simulink library "SignalConditioning_lib"  (Simulink 7.2)
settings: Solver=ode45  SolverMode=SingleTasking  StartTime=0.0  StopTime=10.0  RelTol=1e-3
undefined symbols (not defined in the file or in its folder): ADC, MAG3TempComp, XACCEL, XGYRO, XMAG, YACCEL, YGYRO, YMAG, ZACCEL, ZGYRO, ZMAG
libraries: First_Order_Filter_lib x4, SignalConditioning_lib x3, simulink_extras x2, simulink x1
settings Model: Creator=amurch  LastModifiedBy=lgarbs

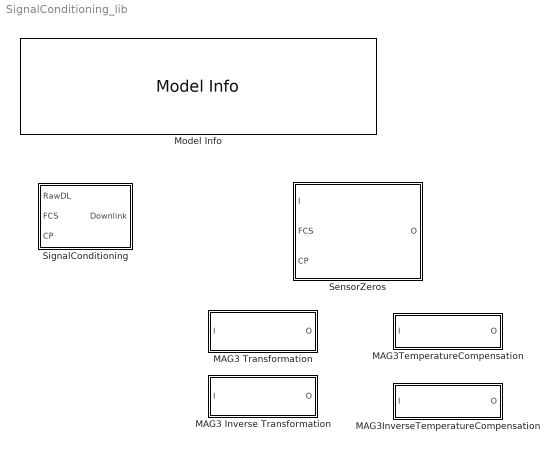
== system SignalConditioning_lib ==
  MAG3 Inverse Transformation : Subsystem
  MAG3 Transformation : Subsystem
  MAG3InverseTemperatureCompensation : Subsystem
  MAG3TemperatureCompensation : Subsystem
  Model Info : simulink/Model-Wide Utilities/Model Info  SystemSampleTime=-1  InitialBlockCM=None  BlockCM=None  Frame=on  DisplayStringWithTags=|  HorizontalTextAlignment=Center  LeftAlignmentValue=0.5  SourceBlockDiagram=SignalConditioning_lib  TagMaxNumber=20
      | Developed using Matlab Release 2007a
      | 
      | SVN:%<ModelVersion>
      | Last modifed by %<LastModifiedBy> on %<LastModificationDate>
  SensorZeros : Subsystem
  SignalConditioning : Subsystem

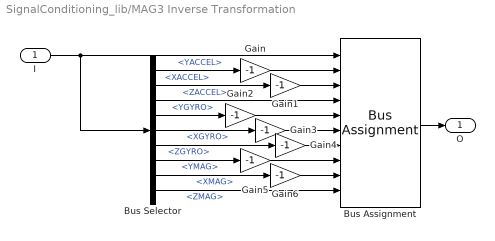
== system SignalConditioning_lib/MAG3 Inverse Transformation ==
  I : Inport  OutDataType=sfix(16)  OutScaling=2^0
  Bus Assignment : BusAssignment  AssignedSignals=XACCEL,YACCEL,ZACCEL,XGYRO,YGYRO,ZGYRO,XMAG,YMAG,ZMAG
  Bus Selector : BusSelector  OutputSignals=YACCEL,XACCEL,ZACCEL,YGYRO,XGYRO,ZGYRO,YMAG,XMAG,ZMAG
  Gain{,1..6} (7 alike) : Gain  Gain=-1  ParameterDataType=sfix(16)  ParameterScaling=2^0  OutDataType=sfix(16)  OutScaling=2^0
  O : Outport  OutDataType=sfix(16)  OutScaling=2^0
  wires:
  Bus Assignment/1 -> O/1
  I/1 -> Bus Assignment/1, Bus Selector/1
  Bus Selector/1 -> Gain/1  "<YACCEL>"
  Gain/1 -> Bus Assignment/2
  Bus Selector/2 -> Gain1/1  "<XACCEL>"
  Bus Selector/3 -> Bus Assignment/4  "<ZACCEL>"
  Gain2/1 -> Bus Assignment/5
  Gain3/1 -> Bus Assignment/6
  Bus Selector/4 -> Gain2/1  "<YGYRO>"
  Bus Selector/5 -> Gain3/1  "<XGYRO>"
  Bus Selector/6 -> Gain4/1  "<ZGYRO>"
  Gain5/1 -> Bus Assignment/8
  Bus Selector/7 -> Gain5/1  "<YMAG>"
  Bus Selector/8 -> Gain6/1  "<XMAG>"
  Bus Selector/9 -> Bus Assignment/10  "<ZMAG>"
  Gain1/1 -> Bus Assignment/3
  Gain4/1 -> Bus Assignment/7
  Gain6/1 -> Bus Assignment/9

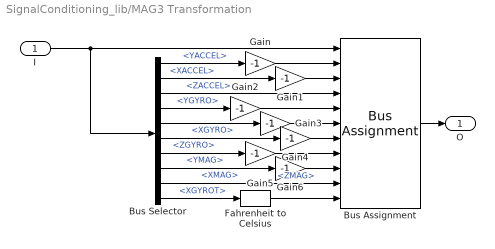
== system SignalConditioning_lib/MAG3 Transformation ==
  I : Inport  OutDataType=sfix(16)  OutScaling=2^0
  Bus Assignment : BusAssignment  AssignedSignals=ADC.XACCEL,ADC.YACCEL,ADC.ZACCEL,ADC.XGYRO,ADC.YGYRO,ADC.ZGYRO,ADC.XMAG,ADC.YMAG,ADC.ZMAG,ADC.XGYROT
  Bus Selector : BusSelector  OutputSignals=ADC.YACCEL,ADC.XACCEL,ADC.ZACCEL,ADC.YGYRO,ADC.XGYRO,ADC.ZGYRO,ADC.YMAG,ADC.XMAG,ADC.ZMAG,ADC.XGYROT
  Fahrenheit to Celsius : simulink_extras/Transformations/Fahrenheit to Celsius  SystemSampleTime=-1
  Gain{,1..6} (7 alike) : Gain  Gain=-1  ParameterDataType=sfix(16)  ParameterScaling=2^0  OutDataType=sfix(16)  OutScaling=2^0
  O : Outport  OutDataType=sfix(16)  OutScaling=2^0
  wires:
  Fahrenheit to Celsius/1 -> Bus Assignment/11
  Bus Selector/10 -> Fahrenheit to Celsius/1  "<XGYROT>"
  I/1 -> Bus Assignment/1, Bus Selector/1
  Bus Assignment/1 -> O/1
  Bus Selector/1 -> Gain/1  "<YACCEL>"
  Gain/1 -> Bus Assignment/2
  Bus Selector/2 -> Gain1/1  "<XACCEL>"
  Gain1/1 -> Bus Assignment/3
  Bus Selector/3 -> Bus Assignment/4  "<ZACCEL>"
  Gain2/1 -> Bus Assignment/5
  Gain3/1 -> Bus Assignment/6
  Bus Selector/4 -> Gain2/1  "<YGYRO>"
  Bus Selector/5 -> Gain3/1  "<XGYRO>"
  Gain4/1 -> Bus Assignment/7
  Bus Selector/6 -> Gain4/1  "<ZGYRO>"
  Gain5/1 -> Bus Assignment/8
  Gain6/1 -> Bus Assignment/9
  Bus Selector/7 -> Gain5/1  "<YMAG>"
  Bus Selector/8 -> Gain6/1  "<XMAG>"
  Bus Selector/9 -> Bus Assignment/10  "<ZMAG>"

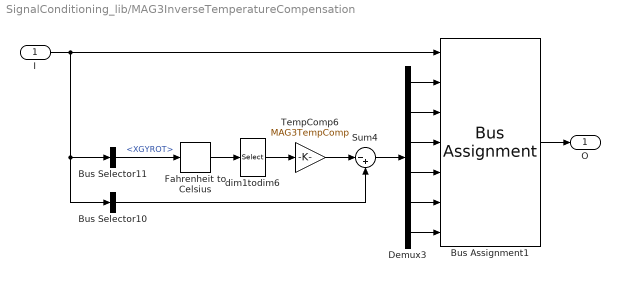
== system SignalConditioning_lib/MAG3InverseTemperatureCompensation ==
  I : Inport  OutDataType=sfix(16)  OutScaling=2^0
  Bus Assignment1 : BusAssignment  AssignedSignals=XGYRO,YGYRO,ZGYRO,XACCEL,YACCEL,ZACCEL
  Bus Selector10 : BusSelector  OutputSignals=XGYRO,YGYRO,ZGYRO,XACCEL,YACCEL,ZACCEL  OutputAsBus=on
  Bus Selector11 : BusSelector  OutputSignals=XGYROT
  Demux3 : Demux  Outputs=6
  Fahrenheit to Celsius : simulink_extras/Transformations/Fahrenheit to Celsius  SystemSampleTime=-1
  Sum4 : Sum  Inputs=|-+  OutDataType=sfix(16)  OutScaling=2^0
  TempComp6 : Gain  Gain=MAG3TempComp  ParameterDataType=sfix(16)  ParameterScaling=2^0  OutDataType=sfix(16)  OutScaling=2^0
  dim1todim6 : Selector  InputPortWidth=1  IndexOptions=Index vector (dialog)  Indices=[1 1 1 1 1 1]  OutputSizes=1
  O : Outport  OutDataType=sfix(16)  OutScaling=2^0
  wires:
  Bus Assignment1/1 -> O/1
  dim1todim6/1 -> TempComp6/1
  Sum4/1 -> Demux3/1
  Demux3/6 -> Bus Assignment1/7
  Demux3/5 -> Bus Assignment1/6
  Demux3/4 -> Bus Assignment1/5
  Demux3/3 -> Bus Assignment1/4
  Demux3/2 -> Bus Assignment1/3
  Demux3/1 -> Bus Assignment1/2
  Bus Selector10/1 -> Sum4/2
  TempComp6/1 -> Sum4/1
  Fahrenheit to Celsius/1 -> dim1todim6/1
  Bus Selector11/1 -> Fahrenheit to Celsius/1  "<XGYROT>"
  I/1 -> Bus Assignment1/1, Bus Selector11/1, Bus Selector10/1

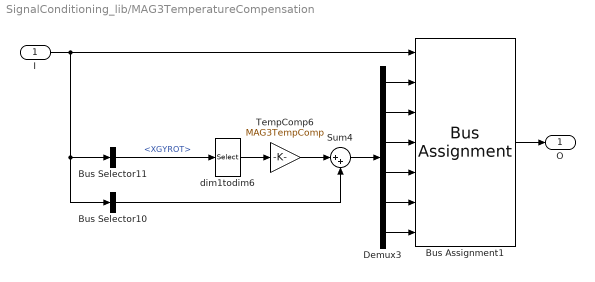
== system SignalConditioning_lib/MAG3TemperatureCompensation ==
  I : Inport  OutDataType=sfix(16)  OutScaling=2^0
  Bus Assignment1 : BusAssignment  AssignedSignals=ADC.XGYRO,ADC.YGYRO,ADC.ZGYRO,ADC.XACCEL,ADC.YACCEL,ADC.ZACCEL
  Bus Selector10 : BusSelector  OutputSignals=ADC.XGYRO,ADC.YGYRO,ADC.ZGYRO,ADC.XACCEL,ADC.YACCEL,ADC.ZACCEL  OutputAsBus=on
  Bus Selector11 : BusSelector  OutputSignals=ADC.XGYROT
  Demux3 : Demux  Outputs=6
  Sum4 : Sum  Inputs=|++  OutDataType=sfix(16)  OutScaling=2^0
  TempComp6 : Gain  Gain=MAG3TempComp  ParameterDataType=sfix(16)  ParameterScaling=2^0  OutDataType=sfix(16)  OutScaling=2^0
  dim1todim6 : Selector  InputPortWidth=1  IndexOptions=Index vector (dialog)  Indices=[1 1 1 1 1 1]  OutputSizes=1
  O : Outport  OutDataType=sfix(16)  OutScaling=2^0
  wires:
  I/1 -> Bus Selector10/1, Bus Selector11/1, Bus Assignment1/1
  Bus Selector11/1 -> dim1todim6/1  "<XGYROT>"
  TempComp6/1 -> Sum4/1
  Bus Selector10/1 -> Sum4/2
  Demux3/1 -> Bus Assignment1/2
  Demux3/2 -> Bus Assignment1/3
  Demux3/3 -> Bus Assignment1/4
  Demux3/4 -> Bus Assignment1/5
  Demux3/5 -> Bus Assignment1/6
  Demux3/6 -> Bus Assignment1/7
  Sum4/1 -> Demux3/1
  dim1todim6/1 -> TempComp6/1
  Bus Assignment1/1 -> O/1

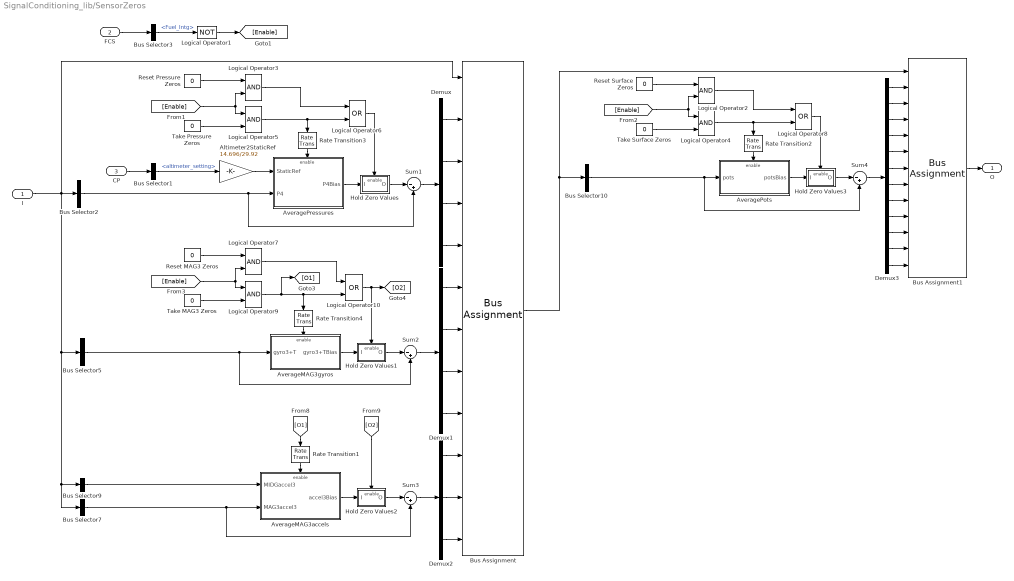
== system SignalConditioning_lib/SensorZeros ==
  I : Inport  OutDataType=sfix(16)  OutScaling=2^0
  FCS : Inport  Port=2  OutDataType=sfix(16)  OutScaling=2^0
  CP : Inport  Port=3  OutDataType=sfix(16)  OutScaling=2^0
  Altimeter2StaticRef : Gain  Gain=14.696/29.92  ParameterDataType=sfix(16)  ParameterScaling=2^0  OutDataType=sfix(16)  OutScaling=2^0
  AverageMAG3accels : Subsystem
  AverageMAG3gyros : Subsystem
  AveragePots : Subsystem
  AveragePressures : Subsystem
  Bus Assignment : BusAssignment  AssignedSignals=ADC.PSL,ADC.PDL,ADC.PSR,ADC.PDR,ADC.XGYRO,ADC.YGYRO,ADC.ZGYRO,ADC.XGYROT,ADC.XACCEL,ADC.YACCEL,ADC.ZACCEL
  Bus Assignment1 : BusAssignment  AssignedSignals=ADC.AILL,ADC.AILR,ADC.FLAPLOB,ADC.FLAPLIB,ADC.FLAPROB,ADC.FLAPRIB,ADC.RUDU,ADC.RUDL,ADC.ELLOB,ADC.ELLIB,ADC.ELROB,ADC.ELRIB
  Bus Selector1 : BusSelector  OutputSignals=CP_constants.altimeter_setting
  Bus Selector10 : BusSelector  OutputSignals=ADC.AILL,ADC.AILR,ADC.FLAPLOB,ADC.FLAPLIB,ADC.FLAPROB,ADC.FLAPRIB,ADC.RUDU,ADC.RUDL,ADC.ELLOB,ADC.ELLIB,ADC.ELROB,ADC.ELRIB  OutputAsBus=on
  Bus Selector2 : BusSelector  OutputSignals=ADC.PSL,ADC.PDL,ADC.PSR,ADC.PDR  OutputAsBus=on
  Bus Selector3 : BusSelector  OutputSignals=RPraw.Fuel_Intg
  Bus Selector5 : BusSelector  OutputSignals=ADC.XGYRO,ADC.YGYRO,ADC.ZGYRO,ADC.XGYROT  OutputAsBus=on
  Bus Selector7 : BusSelector  OutputSignals=ADC.XACCEL,ADC.YACCEL,ADC.ZACCEL  OutputAsBus=on
  Bus Selector9 : BusSelector  OutputSignals=MIDG.MSG_10.nxbody,MIDG.MSG_10.nybody,MIDG.MSG_10.nzbody  OutputAsBus=on
  Demux : Demux
  Demux1 : Demux
  Demux2 : Demux  Outputs=3
  Demux3 : Demux  Outputs=12
  Hold Zero Values : Subsystem  TreatAsAtomicUnit=on
  Hold Zero Values1 : Subsystem  TreatAsAtomicUnit=on
  Hold Zero Values2 : Subsystem  TreatAsAtomicUnit=on
  Hold Zero Values3 : Subsystem  TreatAsAtomicUnit=on
  Logical Operator1 : Logic  Operator=NOT  Inputs=3  AllPortsSameDT=off  OutDataTypeMode=boolean  OutDataTypeStr=boolean
  Logical Operator10 : Logic  Operator=OR  AllPortsSameDT=off  OutDataTypeMode=boolean  OutDataTypeStr=boolean
  Logical Operator{2..5,7,9} (6 alike) : Logic  AllPortsSameDT=off  OutDataTypeMode=boolean  OutDataTypeStr=boolean
  Logical Operator6 : Logic  Operator=OR  AllPortsSameDT=off  OutDataTypeMode=boolean  OutDataTypeStr=boolean
  Logical Operator8 : Logic  Operator=OR  AllPortsSameDT=off  OutDataTypeMode=boolean  OutDataTypeStr=boolean
  Rate Transition{1..4} (4 alike) : RateTransition  Orientation=down  OutPortSampleTime=Timestep
  Reset MAG3 Zeros : Constant  Value=0  OutDataType=sfix(16)  OutScaling=2^0
  Reset Pressure Zeros : Constant  Value=0  OutDataType=sfix(16)  OutScaling=2^0
  Reset Surface Zeros : Constant  Value=0  OutDataType=sfix(16)  OutScaling=2^0
  Sum{1..4} (4 alike) : Sum  Inputs=|-+  OutDataType=sfix(16)  OutScaling=2^0
  Take MAG3 Zeros : Constant  Value=0  OutDataType=sfix(16)  OutScaling=2^0
  Take Pressure Zeros : Constant  Value=0  OutDataType=sfix(16)  OutScaling=2^0
  Take Surface Zeros : Constant  Value=0  OutDataType=sfix(16)  OutScaling=2^0
  O : Outport  OutDataType=sfix(16)  OutScaling=2^0
  wires:
  Logical Operator8/1 -> Hold Zero Values3/Enable
  Logical Operator2/1 -> Logical Operator8/1
  Logical Operator4/1 -> Rate Transition2/1, Logical Operator8/2
  Rate Transition2/1 -> AveragePots/Enable
  [Enable] -> Logical Operator4/1, Logical Operator2/2
  Take Surface Zeros/1 -> Logical Operator4/2
  Reset Surface Zeros/1 -> Logical Operator2/1
  [O2] -> Hold Zero Values2/Enable
  [O1] -> Rate Transition1/1
  Rate Transition1/1 -> AverageMAG3accels/Enable
  Logical Operator7/1 -> Logical Operator10/1
  Logical Operator9/1 -> [O1], Rate Transition4/1, Logical Operator10/2
  [Enable] -> Logical Operator9/1, Logical Operator7/2
  Take MAG3 Zeros/1 -> Logical Operator9/2
  Reset MAG3 Zeros/1 -> Logical Operator7/1
  Logical Operator6/1 -> Hold Zero Values/Enable
  Logical Operator3/1 -> Logical Operator6/1
  Logical Operator5/1 -> Logical Operator6/2, Rate Transition3/1
  Rate Transition3/1 -> AveragePressures/Enable
  [Enable] -> Logical Operator5/1, Logical Operator3/2
  Take Pressure Zeros/1 -> Logical Operator5/2
  Reset Pressure Zeros/1 -> Logical Operator3/1
  Logical Operator10/1 -> [O2], Hold Zero Values1/Enable
  Rate Transition4/1 -> AverageMAG3gyros/Enable
  Logical Operator1/1 -> [Enable]
  FCS/1 -> Bus Selector3/1
  Demux2/3 -> Bus Assignment/12
  Demux2/2 -> Bus Assignment/11
  Demux2/1 -> Bus Assignment/10
  Demux1/4 -> Bus Assignment/9
  Demux1/3 -> Bus Assignment/8
  Demux1/2 -> Bus Assignment/7
  Demux1/1 -> Bus Assignment/6
  Bus Selector9/1 -> AverageMAG3accels/1(MIDGaccel3)
  Bus Selector1/1 -> Altimeter2StaticRef/1  "<altimeter_setting>"
  Altimeter2StaticRef/1 -> AveragePressures/1(StaticRef)
  CP/1 -> Bus Selector1/1
  Bus Selector3/1 -> Logical Operator1/1  "<Fuel_Intg>"
  Hold Zero Values/1(O) -> Sum1/1
  AveragePressures/1(P4Bias) -> Hold Zero Values/1(I)
  Demux/1 -> Bus Assignment/2
  Demux/3 -> Bus Assignment/4
  Bus Selector2/1 -> Sum1/2, AveragePressures/2(P4)
  Sum1/1 -> Demux/1
  Demux/4 -> Bus Assignment/5
  Demux/2 -> Bus Assignment/3
  I/1 -> Bus Selector5/1, Bus Selector9/1, Bus Selector7/1, Bus Selector2/1, Bus Assignment/1
  Hold Zero Values1/1(O) -> Sum2/1
  Sum2/1 -> Demux1/1
  AverageMAG3gyros/1(gyro3+TBias) -> Hold Zero Values1/1(I)
  Bus Selector5/1 -> Sum2/2, AverageMAG3gyros/1(gyro3+T)
  Hold Zero Values2/1(O) -> Sum3/1
  Sum3/1 -> Demux2/1
  AverageMAG3accels/1(accel3Bias) -> Hold Zero Values2/1(I)
  Bus Selector7/1 -> AverageMAG3accels/2(MAG3accel3), Sum3/2
  Hold Zero Values3/1(O) -> Sum4/1
  AveragePots/1(potsBias) -> Hold Zero Values3/1(I)
  Bus Selector10/1 -> AveragePots/1(pots), Sum4/2
  Bus Assignment1/1 -> O/1
  Sum4/1 -> Demux3/1
  Demux3/1 -> Bus Assignment1/2
  Demux3/2 -> Bus Assignment1/3
  Demux3/3 -> Bus Assignment1/4
  Demux3/4 -> Bus Assignment1/5
  Demux3/5 -> Bus Assignment1/6
  Demux3/6 -> Bus Assignment1/7
  Demux3/7 -> Bus Assignment1/8
  Demux3/8 -> Bus Assignment1/9
  Demux3/9 -> Bus Assignment1/10
  Demux3/10 -> Bus Assignment1/11
  Demux3/11 -> Bus Assignment1/12
  Demux3/12 -> Bus Assignment1/13
  Bus Assignment/1 -> Bus Selector10/1, Bus Assignment1/1

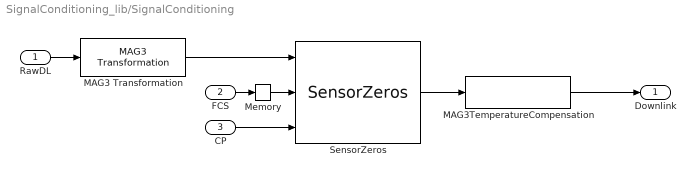
== system SignalConditioning_lib/SignalConditioning ==
  RawDL : Inport  OutDataType=sfix(16)  OutScaling=2^0
  FCS : Inport  Port=2  OutDataType=sfix(16)  OutScaling=2^0
  CP : Inport  Port=3  OutDataType=sfix(16)  OutScaling=2^0
  MAG3 Transformation : SignalConditioning_lib/MAG3 Transformation  SystemSampleTime=-1
  MAG3TemperatureCompensation : SignalConditioning_lib/MAG3TemperatureCompensation  SystemSampleTime=-1
  Memory : Memory
  SensorZeros : SignalConditioning_lib/SensorZeros  SystemSampleTime=-1
  Downlink : Outport  OutDataType=sfix(16)  OutScaling=2^0
  wires:
  Memory/1 -> SensorZeros/2
  CP/1 -> SensorZeros/3
  FCS/1 -> Memory/1
  SensorZeros/1 -> MAG3TemperatureCompensation/1
  MAG3 Transformation/1 -> SensorZeros/1
  RawDL/1 -> MAG3 Transformation/1
  MAG3TemperatureCompensation/1 -> Downlink/1

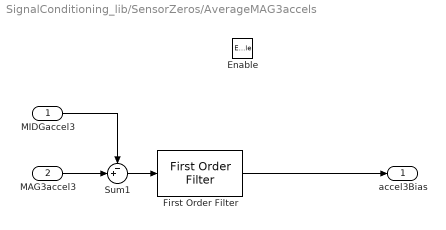
== system SignalConditioning_lib/SensorZeros/AverageMAG3accels ==
  MIDGaccel3 : Inport  OutDataType=sfix(16)  OutScaling=2^0
  MAG3accel3 : Inport  Port=2  OutDataType=sfix(16)  OutScaling=2^0
  Enable : EnablePort
  First Order Filter : First_Order_Filter_lib/First Order Filter  SystemSampleTime=-1  tau=1/pi  timestep=Timestep
  Sum1 : Sum  Inputs=-+|  OutDataType=sfix(16)  OutScaling=2^0
  accel3Bias : Outport  OutDataType=sfix(16)  OutScaling=2^0  OutputWhenDisabled=reset  InitialOutput=[0 0 0]
  wires:
  First Order Filter/1 -> accel3Bias/1
  MIDGaccel3/1 -> Sum1/1
  Sum1/1 -> First Order Filter/1
  MAG3accel3/1 -> Sum1/2

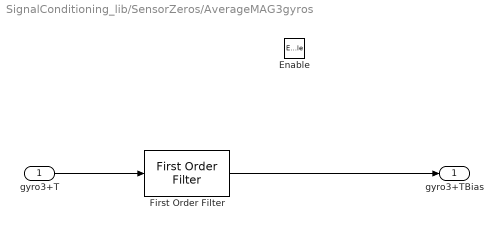
== system SignalConditioning_lib/SensorZeros/AverageMAG3gyros ==
  gyro3+T : Inport  OutDataType=sfix(16)  OutScaling=2^0
  Enable : EnablePort
  First Order Filter : First_Order_Filter_lib/First Order Filter  SystemSampleTime=-1  tau=1/pi  timestep=Timestep
  gyro3+TBias : Outport  OutDataType=sfix(16)  OutScaling=2^0  OutputWhenDisabled=reset  InitialOutput=[0 0 0 0]
  wires:
  gyro3+T/1 -> First Order Filter/1
  First Order Filter/1 -> gyro3+TBias/1

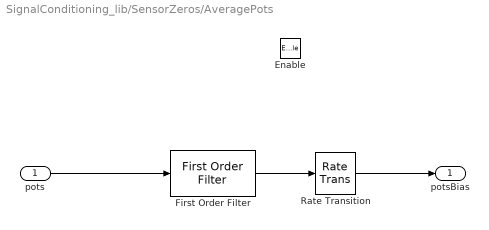
== system SignalConditioning_lib/SensorZeros/AveragePots ==
  pots : Inport  OutDataType=sfix(16)  OutScaling=2^0
  Enable : EnablePort
  First Order Filter : First_Order_Filter_lib/First Order Filter  SystemSampleTime=-1  tau=1/pi  timestep=Timestep
  Rate Transition : RateTransition  Deterministic=off  OutPortSampleTime=Timestep
  potsBias : Outport  OutDataType=sfix(16)  OutScaling=2^0  OutputWhenDisabled=reset  InitialOutput=zeros(1,12)
  wires:
  pots/1 -> First Order Filter/1
  First Order Filter/1 -> Rate Transition/1
  Rate Transition/1 -> potsBias/1

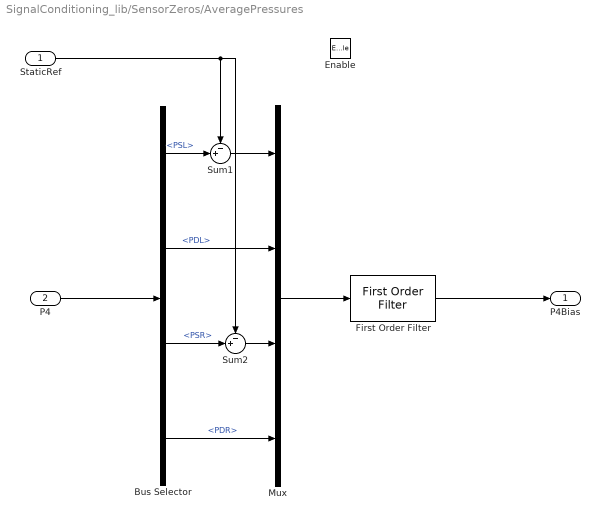
== system SignalConditioning_lib/SensorZeros/AveragePressures ==
  StaticRef : Inport  OutDataType=sfix(16)  OutScaling=2^0
  P4 : Inport  Port=2  OutDataType=sfix(16)  OutScaling=2^0
  Enable : EnablePort
  Bus Selector : BusSelector  OutputSignals=PSL,PDL,PSR,PDR
  First Order Filter : First_Order_Filter_lib/First Order Filter  SystemSampleTime=-1  tau=1/(pi)  timestep=Timestep
  Mux : Mux
  Sum1 : Sum  Inputs=-+|  OutDataType=sfix(16)  OutScaling=2^0
  Sum2 : Sum  Inputs=-+|  OutDataType=sfix(16)  OutScaling=2^0
  P4Bias : Outport  OutDataType=sfix(16)  OutScaling=2^0  OutputWhenDisabled=reset  InitialOutput=[0 0 0 0]
  wires:
  StaticRef/1 -> Sum2/1, Sum1/1
  Bus Selector/3 -> Sum2/2  "<PSR>"
  Sum2/1 -> Mux/3
  Bus Selector/1 -> Sum1/2  "<PSL>"
  Sum1/1 -> Mux/1
  P4/1 -> Bus Selector/1
  Mux/1 -> First Order Filter/1
  Bus Selector/2 -> Mux/2  "<PDL>"
  Bus Selector/4 -> Mux/4  "<PDR>"
  First Order Filter/1 -> P4Bias/1

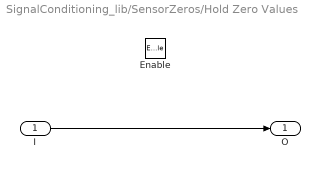
== system SignalConditioning_lib/SensorZeros/Hold Zero Values ==
  I : Inport  OutDataType=sfix(16)  OutScaling=2^0
  Enable : EnablePort
  O : Outport  OutDataType=sfix(16)  OutScaling=2^0
  wires:
  I/1 -> O/1

== system SignalConditioning_lib/SensorZeros/Hold Zero Values1 ==
  I : Inport  OutDataType=sfix(16)  OutScaling=2^0
  Enable : EnablePort
  O : Outport  OutDataType=sfix(16)  OutScaling=2^0
  wires:
  I/1 -> O/1

== system SignalConditioning_lib/SensorZeros/Hold Zero Values2 ==
  I : Inport  OutDataType=sfix(16)  OutScaling=2^0
  Enable : EnablePort
  O : Outport  OutDataType=sfix(16)  OutScaling=2^0
  wires:
  I/1 -> O/1

== system SignalConditioning_lib/SensorZeros/Hold Zero Values3 ==
  I : Inport  OutDataType=sfix(16)  OutScaling=2^0
  Enable : EnablePort
  O : Outport  OutDataType=sfix(16)  OutScaling=2^0
  wires:
  I/1 -> O/1
